simulink model "Lab1Exp2"  (R2021a)
settings: Solver=VariableStepAuto  StartTime=0.0  StopTime=10.0  RelTol=1e-3
values from neighbouring files (symbols this model uses):
  denC1 = 1    [Lab1Teste2.m]
  denC2 = (1/(R*C)+Po/(C*Vc0^2)+rl/L)    (= 145.202020202)    [Lab1Teste2.m]
  denC3 = ((Po*rl/Vc0^2+rl/R+1)*1/(L*C))    (= 454545.454545)    [Lab1Teste2.m]
  H = 1    [Lab1Teste2.m]
  numFT = Vin/(C*L)    (= 9090909.09091)    [Lab1Teste2.m]
settings Model: Creator=DaniSan  LastModifiedBy=DaniSan

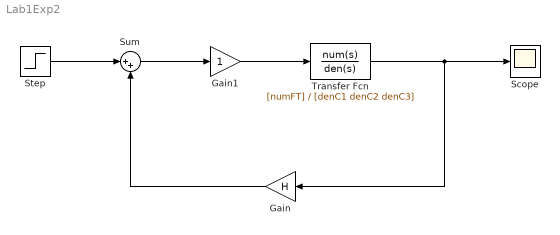
== system Lab1Exp2 ==
  Gain : Gain  Gain=H
  Gain1 : Gain
  Scope : Scope
  Step : Step  SampleTime=0
  Sum : Sum  Inputs=|++
  Transfer Fcn : TransferFcn  Numerator=[numFT]  Denominator=[denC1 denC2 denC3]
  wires:
  Step/1 -> Sum/1
  Transfer Fcn/1 -> Gain/1, Scope/1
  Gain/1 -> Sum/2
  Sum/1 -> Gain1/1
  Gain1/1 -> Transfer Fcn/1
